simulink model "DDK_DCSUV_50ms_2020a"  (R2021a)
settings: Solver=VariableStepAuto  StartTime=0.0  StopTime=inf  FixedStep=0.001  RelTol=1e-3
libraries: Solver_SF x1
settings Model: Creator=no_en  LastModifiedBy=Administrator
settings SolverCC: AlgebraicLoopSolver=TrustRegion
settings DataIOCC: SaveState=on  ReturnWorkspaceOutputs=off
settings DebuggingCC: SFMachineParentedDataDiag=warning  ArithmeticOperatorsInVariantConditions=warning
settings SFSimCC: SimUseLocalCustomCode=off  CustomCodeUndefinedFunction=UseInterfaceOnly
settings RTWCC: RTWUseLocalCustomCode=off

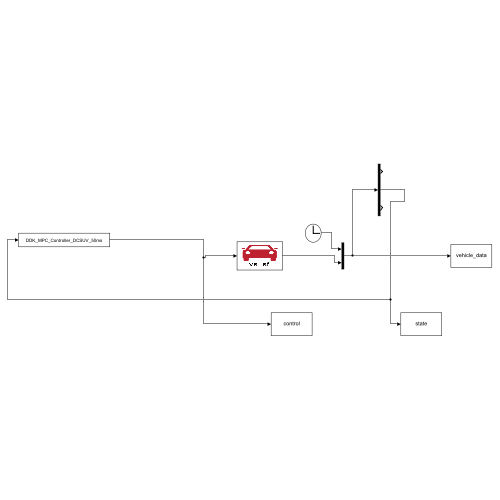
[thumbnail: Simulink's stored preview of the top-level diagram]
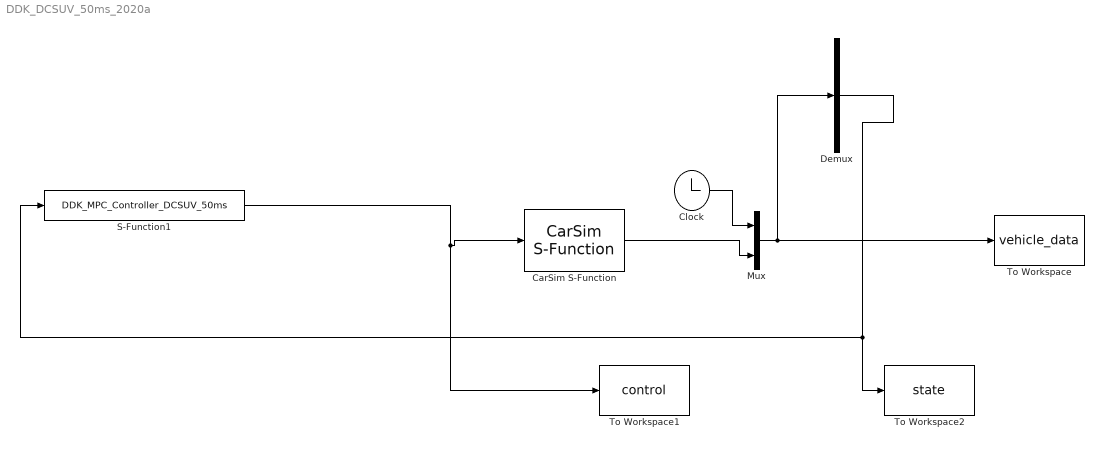
== system DDK_DCSUV_50ms_2020a ==
  CarSim S-Function : Solver_SF/CarSim S-Function  Priority=1  SIMFILE=simfile.sim
  Clock : Clock
  Demux : Demux  Outputs=[1 6 7]
  Mux : Mux  Inputs=2
  S-Function1 : S-Function  FunctionName=DDK_MPC_Controller_DCSUV_50ms  SFunctionDeploymentMode=off  EnableBusSupport=off
  To Workspace : ToWorkspace  VariableName=vehicle_data  SaveFormat=Timeseries  SampleTime=0.01
  To Workspace1 : ToWorkspace  VariableName=control  SaveFormat=Timeseries  SampleTime=0.01
  To Workspace2 : ToWorkspace  VariableName=state  SaveFormat=Timeseries  SampleTime=0.01
  wires:
  Clock/1 -> Mux/1
  CarSim S-Function/1 -> Mux/2
  Mux/1 -> Demux/1, To Workspace/1
  Demux/2 -> S-Function1/1, To Workspace2/1
  S-Function1/1 -> To Workspace1/1, CarSim S-Function/1
